simulink model "plant_uncontrolled"  (R2024b)
settings: Solver=VariableStepAuto  StartTime=0.0  StopTime=t_sim  MaxStep=0.001  RelTol=1e-3
values from neighbouring files (symbols this model uses):
  b = 0.0245    [Main_uncontrolled.m]
  data_sys = [m r g J b lx ly]    [Main_uncontrolled.m]
  lx = 0.182    [Main_uncontrolled.m]
  ly = 0.150    (= 0.15)    [Main_uncontrolled.m]
  zx0 = [x0 xp0]'    [Main_uncontrolled.m]
  zy0 = [y0 yp0]'    [Main_uncontrolled.m]
settings Model: Creator=nicvi  LastModifiedBy=nicvi

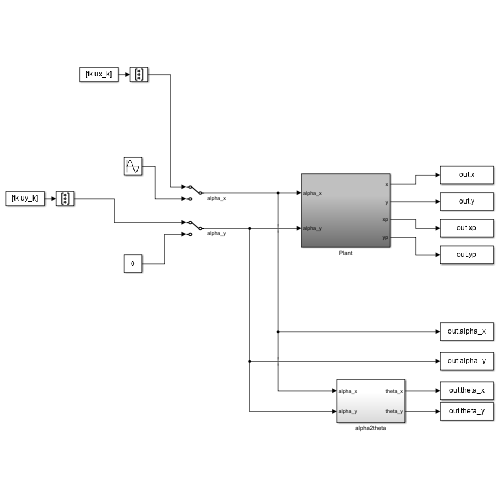
[thumbnail: Simulink's stored preview of the top-level diagram]
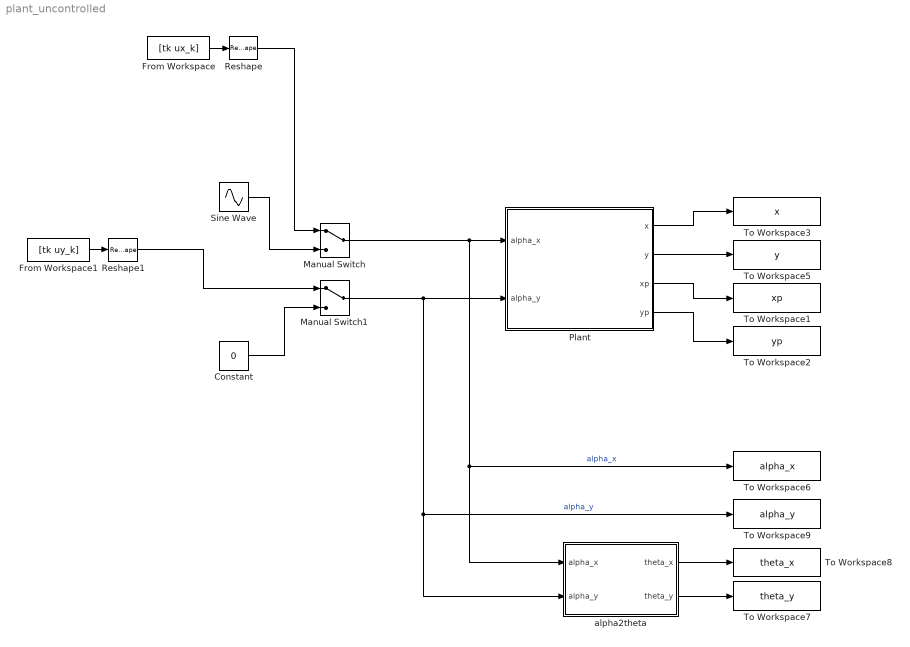
== system plant_uncontrolled ==
  Constant : Constant  Value=0  SampleTime=-1
  From Workspace : FromWorkspace  VariableName=[tk ux_k]
  From Workspace1 : FromWorkspace  VariableName=[tk uy_k]
  Manual Switch : ManualSwitch
  Manual Switch1 : ManualSwitch
  Plant : Subsystem
  Reshape : Reshape  OutputDimensionality=Column vector (2-D)
  Reshape1 : Reshape  OutputDimensionality=Column vector (2-D)
  Sine Wave : Sin  Amplitude=deg2rad(15)  Frequency=5  SampleTime=0
  To Workspace1 : ToWorkspace  VariableName=xp  SampleTime=-1
      settings: Save2DSignal=2-D array (concatenate along first dimension)
  To Workspace2 : ToWorkspace  VariableName=yp  SampleTime=-1
      settings: Save2DSignal=2-D array (concatenate along first dimension)
  To Workspace3 : ToWorkspace  VariableName=x  SampleTime=-1
      settings: Save2DSignal=2-D array (concatenate along first dimension)
  To Workspace5 : ToWorkspace  VariableName=y  SampleTime=-1
      settings: Save2DSignal=2-D array (concatenate along first dimension)
  To Workspace6 : ToWorkspace  VariableName=alpha_x  SampleTime=-1
      settings: Save2DSignal=2-D array (concatenate along first dimension)
  To Workspace7 : ToWorkspace  VariableName=theta_y  SampleTime=-1
      settings: Save2DSignal=2-D array (concatenate along first dimension)
  To Workspace8 : ToWorkspace  VariableName=theta_x  SampleTime=-1
      settings: Save2DSignal=2-D array (concatenate along first dimension)
  To Workspace9 : ToWorkspace  VariableName=alpha_y  SampleTime=-1
      settings: Save2DSignal=2-D array (concatenate along first dimension)
  alpha2theta : Subsystem
  wires:
  Constant/1 -> Manual Switch1/2
  Manual Switch/1 -> Plant/1(alpha_x), To Workspace6/1, alpha2theta/1(alpha_x)  "alpha_x"
  Manual Switch1/1 -> Plant/2(alpha_y), To Workspace9/1, alpha2theta/2(alpha_y)  "alpha_y"
  Sine Wave/1 -> Manual Switch/2
  Plant/1(x) -> To Workspace3/1
  Plant/2(y) -> To Workspace5/1
  alpha2theta/2(theta_y) -> To Workspace7/1
  alpha2theta/1(theta_x) -> To Workspace8/1
  From Workspace/1 -> Reshape/1
  Reshape/1 -> Manual Switch/1
  From Workspace1/1 -> Reshape1/1
  Reshape1/1 -> Manual Switch1/1
  Plant/3(xp) -> To Workspace1/1
  Plant/4(yp) -> To Workspace2/1

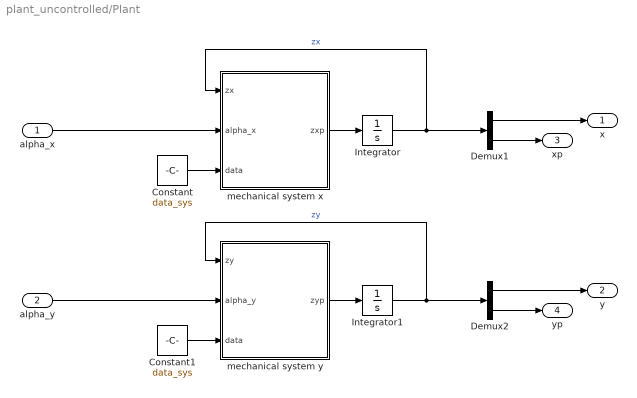
== system plant_uncontrolled/Plant ==
  alpha_x : Inport
  alpha_y : Inport  Port=2
  Constant : Constant  Value=data_sys
  Constant1 : Constant  Value=data_sys
  Demux1 : Demux  Outputs=2
  Demux2 : Demux  Outputs=2
  Integrator : Integrator  InitialCondition=zx0
  Integrator1 : Integrator  InitialCondition=zy0
  mechanical system x : MATLAB Function  TreatAsAtomicUnit=on
  mechanical system y : MATLAB Function  TreatAsAtomicUnit=on
  x : Outport
  y : Outport  Port=2
  xp : Outport  Port=3
  yp : Outport  Port=4
  wires:
  mechanical system x/1(zxp) -> Integrator/1
  Integrator/1 -> Demux1/1, mechanical system x/1(zx)  "zx"
  Constant/1 -> mechanical system x/3(data)
  Constant1/1 -> mechanical system y/3(data)
  mechanical system y/1(zyp) -> Integrator1/1
  Integrator1/1 -> mechanical system y/1(zy), Demux2/1  "zy"
  Demux1/1 -> x/1
  Demux1/2 -> xp/1
  Demux2/2 -> yp/1
  Demux2/1 -> y/1
  alpha_x/1 -> mechanical system x/2(alpha_x)
  alpha_y/1 -> mechanical system y/2(alpha_y)

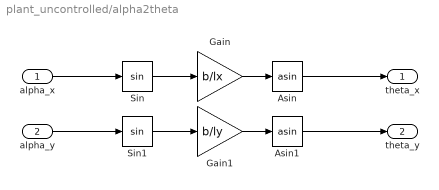
== system plant_uncontrolled/alpha2theta ==
  alpha_x : Inport
  alpha_y : Inport  Port=2
  Asin : Trigonometry  Operator=asin
  Asin1 : Trigonometry  Operator=asin
  Gain : Gain  Gain=b/lx
  Gain1 : Gain  Gain=b/ly
  Sin : Trigonometry
  Sin1 : Trigonometry
  theta_x : Outport
  theta_y : Outport  Port=2
  wires:
  Gain/1 -> Asin/1
  Sin1/1 -> Gain1/1
  alpha_y/1 -> Sin1/1
  Sin/1 -> Gain/1
  Asin1/1 -> theta_y/1
  Gain1/1 -> Asin1/1
  Asin/1 -> theta_x/1
  alpha_x/1 -> Sin/1

== matlab function plant_uncontrolled/Plant/mechanical system x ==
  data: zx input; alpha_x input; zxp output; data input
function zxp=fcn(zx,alpha_x,data)

% extract data

m=data(1); 
r=data(2);
g=data(3);
J=data(4);
b=data(5);
lx=data(6);

% equation of motion

zxp=zeros(2,1);

zxp(1) = zx(2);
zxp(2) = (m*g*b) / (lx*(m+J/r^2)) * sin(alpha_x);

end

== matlab function plant_uncontrolled/Plant/mechanical system y ==
  data: zy input; alpha_y input; zyp output; data input
function zyp=fcn(zy,alpha_y,data)

% extract data

m=data(1); 
r=data(2);
g=data(3);
J=data(4);
b=data(5);
ly=data(7);

% equation of motion

zyp=zeros(2,1);

zyp(1) = zy(2);
zyp(2) = (m*g*b) / (ly*(m+J/r^2)) * sin(alpha_y);

end
